simulink model "open_loop"  (R2018b)
settings: Solver=VariableStepAuto  StartTime=0.0  StopTime=10.0  RelTol=1e-3
settings Model: Creator=LEGION  LastModifiedBy=LEGION

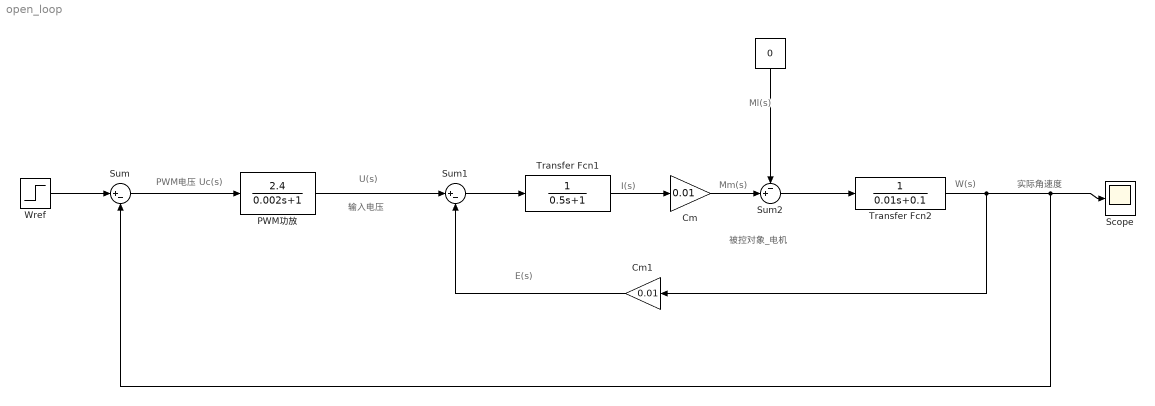
== system open_loop ==
  note: 被控对象_电机
  note: W(s)
  note: I(s)
  note: Mm(s)
  note: 实际角速度
  note: Ml(s)
  note: E(s)
  note: 输入电压
  note: U(s)
  note: PWM电压 Uc(s)
  " " : Constant  Value=0
  Cm : Gain  Gain=0.01
  Cm1 : Gain  Gain=0.01
  PWM功放 : TransferFcn  Numerator=[2.4]  Denominator=[0.002 1]
  Scope : Scope
  Sum : Sum  Inputs=|+-
  Sum1 : Sum  Inputs=|+-
  Sum2 : Sum  Inputs=-+|
  Transfer Fcn1 : TransferFcn  Denominator=[0.5 1]
  Transfer Fcn2 : TransferFcn  Denominator=[0.01 0.1]
  Wref : Step  Time=0  SampleTime=0
  wires:
  PWM功放/1 -> Sum1/1
  Sum1/1 -> Transfer Fcn1/1
  Cm/1 -> Sum2/2
  Transfer Fcn2/1 -> Sum/2, Scope/1, Cm1/1
  " "/1 -> Sum2/1
  Cm1/1 -> Sum1/2
  Sum2/1 -> Transfer Fcn2/1
  Transfer Fcn1/1 -> Cm/1
  Wref/1 -> Sum/1
  Sum/1 -> PWM功放/1
